simulink model "Bioloid_DFK_MDL_SV"  (R2013a)
settings: Solver=ode45  StartTime=0.0  StopTime=20  FixedStep=0.001  RelTol=1e-12
undefined symbols (not defined in the file or in its folder): Bioloid_DFK_SV, Bioloid_Ja_SV, Bioloid_Jg_SV, Bioloid_Signals2VRML, Error_Poses, ToSimulink_Bioloid_FK_ST
libraries: simulink x24, vrlib x1
settings Model: Creator=Jose Angel Rangel  LastModifiedBy=Angel

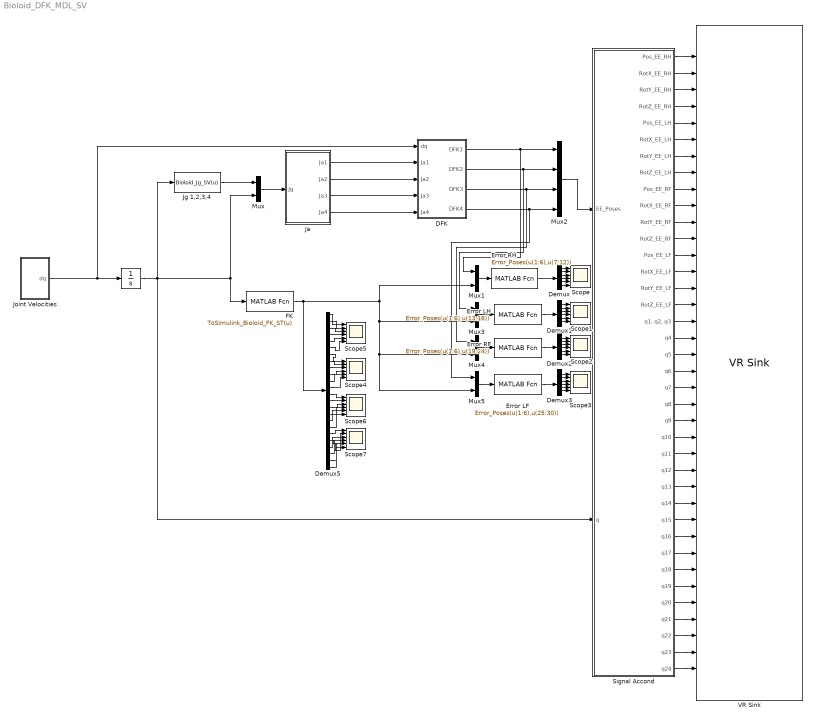
== system Bioloid_DFK_MDL_SV ==
  " " : Integrator
  DFK : Subsystem
  Demux{,1..3} (4 alike) : Demux  Outputs=6
  Demux5 : Demux  Outputs=24
  Error LF : MATLABFcn  MATLABFcn=Error_Poses(u(1:6),u(25:30))  OutputDimensions=6
  Error LH : MATLABFcn  MATLABFcn=Error_Poses(u(1:6),u(13:18))  OutputDimensions=6
  Error RF : MATLABFcn  MATLABFcn=Error_Poses(u(1:6),u(19:24))  OutputDimensions=6
  Error RH : MATLABFcn  MATLABFcn=Error_Poses(u(1:6),u(7:12))  OutputDimensions=6
  FK : MATLABFcn  MATLABFcn=ToSimulink_Bioloid_FK_ST(u)  OutputDimensions=24
  "Ja " : Subsystem
  Jg 1,2,3,4 : MATLABFcn  MATLABFcn=Bioloid_Jg_SV(u)  OutputDimensions=600
  Joint Velocities : Subsystem
  Mux{,1,3..5} (5 alike) : Mux  Inputs=2
  Mux2 : Mux
  Scope{,1..7} (8 alike) : Scope  NumInputPorts=6
      Scope settings: YMin=7e-10~1.03398e-25~0~-1~-1~-7e-06  YMax=1.7e-09~2.75e-09~6e-17~1~1~-1e-06
      Scope1 settings: TimeRange=10  YMin=-2.5e-05~-5e-06~-2e-05~-1~-0.007~-7  YMax=5e-06~3.5e-05~2.5e-06~7~0.001~1
      Scope2 settings: YMin=-7e-05~-0.000175~-2e-05~-5~-0.075~-3.5  YMax=1e-05~2.5e-05~6e-05~40~0.1~0.5  SaveName=ScopeData2
      Scope3 settings: YMin=-7e-05~-0.000175~-2e-05~-5~-0.075~-3.5  YMax=1e-05~2.5e-05~6e-05~40~0.1~0.5  SaveName=ScopeData3
      Scope4 settings: YMin=-2e-05~-9e-05~4e-05~0~-0.015~-7  YMax=7.5e-06~-2e-05~0.00011~7~-0.005~0  SaveName=ScopeData4
      Scope5 settings: YMin=4.6~4.6~4.9~-1.7~-0.015~-7  YMax=5.6~5.4~5.8~-0.7~-0.005~0  SaveName=ScopeData5
      Scope6 settings: YMin=-2e-05~-9e-05~4e-05~0~-0.015~-7  YMax=7.5e-06~-2e-05~0.00011~7~-0.005~0  SaveName=ScopeData6
      Scope7 settings: YMin=-2e-05~-9e-05~4e-05~0~-0.015~-7  YMax=7.5e-06~-2e-05~0.00011~7~-0.005~0  SaveName=ScopeData7
  Signal Accond : Subsystem
  VR Sink : vrlib/VR Sink  InstantiateOnLoad=on  SampleTime=0.1  ViewEnable=on  RemoteChange=off  RemoteView=off  FieldsWritten=EE_RH_Traslation.translation.3.1.1.double#EE_RH_RotX.rotation.4.1.1.double#EE_RH_RotY.rotation.4.1.1.double#EE_RH_RotZ.rotation.4.1.1.double#EE_LH_Traslation.translation.3.1.1.double#EE_LH_RotX.rotation.4.1.1.double#EE_LH_RotY.rotation.4.1.1.double#EE_LH_RotZ.rotation.4.1.1.double#EE_RF_Traslation.translation.3.1.1.double#EE_RF_RotX.rotation.4.1.1.double#EE_RF_RotY.rotation.4.1.1.double#EE_RF_RotZ.rotation.4.1.1.double#EE_LF_Traslation.translation.3.1.1.double#EE_LF_RotX.rotation.4.1.1.double#EE_LF_RotY.rotation.4.1.1.double#EE_LF_RotZ.rotation.4.1.1.double#TrunkTraslation.translation.3.1.1.double#TrunkRotX.rotation.4.1.1.double#TrunkRotY.rotation.4.1.1.double#TrunkRotZ.rotation.4.1.1.double#Right_Arm.rotation.4.1.1.double#Right_Humeros1.rotation.4.1.1.double#Right_Hand1.rotation.4.1.1.double#Left_Arm.rotation.4.1.1.double#Left_Humeros1.rotation.4.1.1.double#Left_Hand1.rotation.4.1.1.double#Right_Groin.rotation.4.1.1.double#Right_Hip1.rotation.4.1.1.double#Right_Femur1.rotation.4.1.1.double#Right_Tibia1.rotation.4.1.1.double#Right_Ankle1.rotation.4.1.1.double#Right_Foot1.rotation.4.1.1.double#Left_Groin.rotation.4.1.1.double#Left_Hip1.rotation.4.1.1.double#Left_Femur1.rotation.4.1.1.double#Left_Tibia1.rotation.4.1.1.double#Left_Ankle1.rotation.4.1.1.double#Left_Foot1.rotation.4.1.1.double  WorldFileName=Bioloid (Fisico White_Background).WRL  AutoView=off  VideoDimensions=[]  AllowVariableSize=off
  wires:
  Jg 1,2,3,4/1 -> Mux/1
  "Ja "/1(Ja1) -> DFK/2(Ja1)
  "Ja "/2(Ja2) -> DFK/3(Ja2)
  "Ja "/3(Ja3) -> DFK/4(Ja3)
  "Ja "/4(Ja4) -> DFK/5(Ja4)
  Joint Velocities/1(dq) -> DFK/1(dq), " "/1
  " "/1 -> Signal Accond/2(q), Mux/2, FK/1, Jg 1,2,3,4/1
  DFK/1(DFK1) -> Mux1/1, Mux2/1
  DFK/2(DFK2) -> Mux3/1, Mux2/2
  DFK/3(DFK3) -> Mux4/1, Mux2/3
  DFK/4(DFK4) -> Mux5/1, Mux2/4
  Demux/6 -> Scope/6
  Demux/3 -> Scope/3
  Demux/4 -> Scope/4
  Demux/5 -> Scope/5
  Demux/2 -> Scope/2
  Demux/1 -> Scope/1
  Demux1/6 -> Scope1/6
  Demux1/3 -> Scope1/3
  Demux1/4 -> Scope1/4
  Demux1/5 -> Scope1/5
  Demux1/2 -> Scope1/2
  Demux1/1 -> Scope1/1
  Demux2/6 -> Scope2/6
  Demux2/3 -> Scope2/3
  Demux2/4 -> Scope2/4
  Demux2/5 -> Scope2/5
  Demux2/2 -> Scope2/2
  Demux2/1 -> Scope2/1
  Demux3/6 -> Scope3/6
  Demux3/3 -> Scope3/3
  Demux3/4 -> Scope3/4
  Demux3/5 -> Scope3/5
  Demux3/2 -> Scope3/2
  Demux3/1 -> Scope3/1
  Mux1/1 -> Error RH/1
  Mux3/1 -> Error LH/1
  Mux4/1 -> Error RF/1
  Mux5/1 -> Error LF/1
  Error RH/1 -> Demux/1
  Mux/1 -> "Ja "/1(Jg)
  Error LH/1 -> Demux1/1
  Error RF/1 -> Demux2/1
  Error LF/1 -> Demux3/1
  Signal Accond/1(Pos_EE_RH) -> VR Sink/1
  Signal Accond/2(RotX_EE_RH) -> VR Sink/2
  Signal Accond/3(RotY_EE_RH) -> VR Sink/3
  Signal Accond/4(RotZ_EE_RH) -> VR Sink/4
  Signal Accond/5(Pos_EE_LH) -> VR Sink/5
  Signal Accond/30(q16) -> VR Sink/30
  Signal Accond/16(RotZ_EE_LF) -> VR Sink/16
  Signal Accond/36(q22) -> VR Sink/36
  Signal Accond/24(q10) -> VR Sink/24
  Signal Accond/22(q8) -> VR Sink/22
  Signal Accond/31(q17) -> VR Sink/31
  Signal Accond/20(q6) -> VR Sink/20
  Signal Accond/32(q18) -> VR Sink/32
  Signal Accond/21(q7) -> VR Sink/21
  Signal Accond/6(RotX_EE_LH) -> VR Sink/6
  Signal Accond/7(RotY_EE_LH) -> VR Sink/7
  Signal Accond/18(q4) -> VR Sink/18
  Signal Accond/25(q11) -> VR Sink/25
  Signal Accond/26(q12) -> VR Sink/26
  Signal Accond/15(RotY_EE_LF) -> VR Sink/15
  Signal Accond/38(q24) -> VR Sink/38
  Signal Accond/17("q1, q2, q3") -> VR Sink/17
  Signal Accond/29(q15) -> VR Sink/29
  Signal Accond/9(Pos_EE_RF) -> VR Sink/9
  Signal Accond/27(q13) -> VR Sink/27
  Signal Accond/10(RotX_EE_RF) -> VR Sink/10
  Signal Accond/12(RotZ_EE_RF) -> VR Sink/12
  Signal Accond/8(RotZ_EE_LH) -> VR Sink/8
  Signal Accond/19("q5 ") -> VR Sink/19
  Signal Accond/13(Pos_EE_LF) -> VR Sink/13
  Signal Accond/33(q19) -> VR Sink/33
  Signal Accond/35(q21) -> VR Sink/35
  Signal Accond/11(RotY_EE_RF) -> VR Sink/11
  Signal Accond/34(q20) -> VR Sink/34
  Signal Accond/14(RotX_EE_LF) -> VR Sink/14
  Signal Accond/23(q9) -> VR Sink/23
  Signal Accond/28(q14) -> VR Sink/28
  Signal Accond/37(q23) -> VR Sink/37
  Mux2/1 -> Signal Accond/1(EE_Poses)
  FK/1 -> Demux5/1, Mux3/2, Mux5/2, Mux4/2, Mux1/2
  Demux5/1 -> Scope5/1
  Demux5/2 -> Scope5/2
  Demux5/3 -> Scope5/3
  Demux5/4 -> Scope5/4
  Demux5/5 -> Scope5/5
  Demux5/6 -> Scope5/6
  Demux5/7 -> Scope4/1
  Demux5/8 -> Scope4/2
  Demux5/9 -> Scope4/3
  Demux5/10 -> Scope4/4
  Demux5/11 -> Scope4/5
  Demux5/12 -> Scope4/6
  Demux5/13 -> Scope6/1
  Demux5/14 -> Scope6/2
  Demux5/15 -> Scope6/3
  Demux5/16 -> Scope6/4
  Demux5/17 -> Scope6/5
  Demux5/18 -> Scope6/6
  Demux5/19 -> Scope7/1
  Demux5/20 -> Scope7/2
  Demux5/21 -> Scope7/3
  Demux5/22 -> Scope7/4
  Demux5/23 -> Scope7/5
  Demux5/24 -> Scope7/6

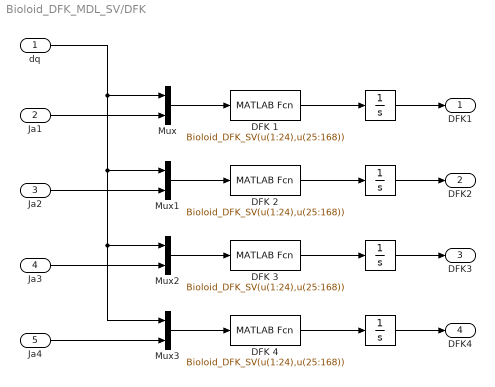
== system Bioloid_DFK_MDL_SV/DFK ==
  dq : Inport
  Ja1 : Inport  Port=2
  Ja2 : Inport  Port=3
  Ja3 : Inport  Port=4
  Ja4 : Inport  Port=5
  "  " : Integrator  InitialCondition=[0;-0.2250;-0.0145;0;0;0]
  "    " : Integrator  InitialCondition=[0;0.225;-0.0145;0;0;0]
  "     " : Integrator  InitialCondition=[0;-0.0385;-0.30250;0;0;0]
  "      " : Integrator  InitialCondition=[0;0.0385;-0.3025;0;0;0]
  DFK {1..4} (4 alike) : MATLABFcn  MATLABFcn=Bioloid_DFK_SV(u(1:24),u(25:168))  OutputDimensions=6
  Mux{,1..3} (4 alike) : Mux  Inputs=2
  DFK1 : Outport
  DFK2 : Outport  Port=2
  DFK3 : Outport  Port=3
  DFK4 : Outport  Port=4
  wires:
  DFK 1/1 -> "  "/1
  DFK 2/1 -> "    "/1
  DFK 3/1 -> "     "/1
  DFK 4/1 -> "      "/1
  dq/1 -> Mux3/1, Mux2/1, Mux1/1, Mux/1
  Mux/1 -> DFK 1/1
  Mux1/1 -> DFK 2/1
  Mux2/1 -> DFK 3/1
  Mux3/1 -> DFK 4/1
  Ja1/1 -> Mux/2
  Ja2/1 -> Mux1/2
  Ja3/1 -> Mux2/2
  Ja4/1 -> Mux3/2
  "  "/1 -> DFK1/1
  "    "/1 -> DFK2/1
  "     "/1 -> DFK3/1
  "      "/1 -> DFK4/1

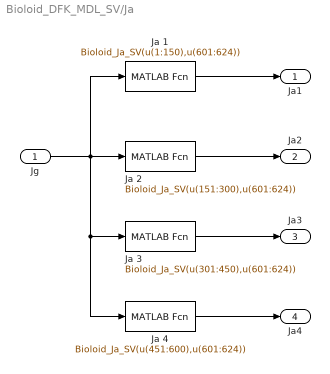
== system Bioloid_DFK_MDL_SV/Ja  ==
  Jg : Inport
  Ja 1 : MATLABFcn  MATLABFcn=Bioloid_Ja_SV(u(1:150),u(601:624))  OutputDimensions=144
  Ja 2 : MATLABFcn  MATLABFcn=Bioloid_Ja_SV(u(151:300),u(601:624))  OutputDimensions=144
  Ja 3 : MATLABFcn  MATLABFcn=Bioloid_Ja_SV(u(301:450),u(601:624))  OutputDimensions=144
  Ja 4 : MATLABFcn  MATLABFcn=Bioloid_Ja_SV(u(451:600),u(601:624))  OutputDimensions=144
  Ja1 : Outport
  Ja2 : Outport  Port=2
  Ja3 : Outport  Port=3
  Ja4 : Outport  Port=4
  wires:
  Jg/1 -> Ja 1/1, Ja 2/1, Ja 3/1, Ja 4/1
  Ja 4/1 -> Ja4/1
  Ja 1/1 -> Ja1/1
  Ja 3/1 -> Ja3/1
  Ja 2/1 -> Ja2/1

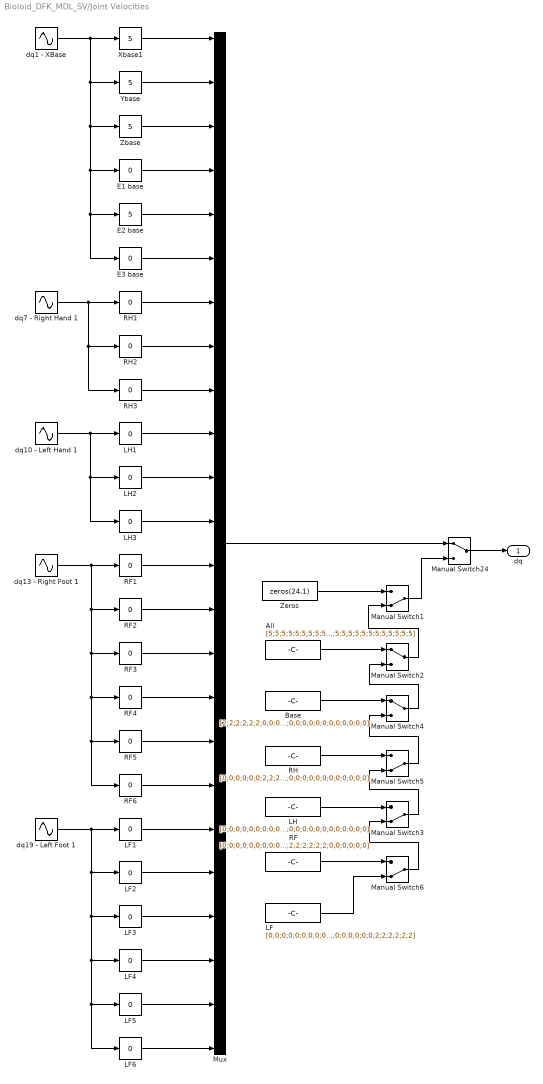
== system Bioloid_DFK_MDL_SV/Joint Velocities ==
  All : Constant  Value=[5;5;5;5;5;5;5;5;5;5;5;5;5;5;5;5;5;5;5;5;5;5;5;5]
  Base : Constant  Value=[2;2;2;2;2;2;0;0;0;0;0;0;0;0;0;0;0;0;0;0;0;0;0;0]
  E1 base : simulink/Math Operations/Slider Gain  low=-5  gain=0  high=5
  E2 base : simulink/Math Operations/Slider Gain  low=-5  gain=5  high=5
  E3 base : simulink/Math Operations/Slider Gain  low=-5  gain=0  high=5
  LF : Constant  Value=[0;0;0;0;0;0;0;0;0;0;0;0;0;0;0;0;0;0;2;2;2;2;2;2]
  LF{1..6} (6 alike) : simulink/Math Operations/Slider Gain  low=0  gain=0  high=5
  LH : Constant  Value=[0;0;0;0;0;0;0;0;0;2;2;2;0;0;0;0;0;0;0;0;0;0;0;0]
  LH1 : simulink/Math Operations/Slider Gain  low=0  gain=0  high=5
  LH2 : simulink/Math Operations/Slider Gain  low=0  gain=0  high=5
  LH3 : simulink/Math Operations/Slider Gain  low=0  gain=0  high=5
  Manual Switch{1,3,5..6} (4 alike) : ManualSwitch  CurrentSetting=0
  Manual Switch2 : ManualSwitch
  Manual Switch24 : ManualSwitch
  Manual Switch4 : ManualSwitch
  Mux : Mux  Inputs=24
  RF : Constant  Value=[0;0;0;0;0;0;0;0;0;0;0;0;2;2;2;2;2;2;0;0;0;0;0;0]
  RF{1..6} (6 alike) : simulink/Math Operations/Slider Gain  low=0  gain=0  high=5
  RH : Constant  Value=[0;0;0;0;0;0;2;2;2;0;0;0;0;0;0;0;0;0;0;0;0;0;0;0]
  RH1 : simulink/Math Operations/Slider Gain  low=0  gain=0  high=5
  RH2 : simulink/Math Operations/Slider Gain  low=0  gain=0  high=5
  RH3 : simulink/Math Operations/Slider Gain  low=0  gain=0  high=5
  Xbase1 : simulink/Math Operations/Slider Gain  low=-5  gain=5  high=5
  Ybase : simulink/Math Operations/Slider Gain  low=-5  gain=5  high=5
  Zbase : simulink/Math Operations/Slider Gain  low=-5  gain=5  high=5
  Zeros : Constant  Value=zeros(24,1)
  dq1 - XBase : Sin  SampleTime=0
  dq10 - Left Hand 1 : Sin  SampleTime=0
  dq13 - Right Foot 1 : Sin  SampleTime=0
  dq19 - Left Foot 1 : Sin  SampleTime=0
  dq7 - Right Hand 1 : Sin  SampleTime=0
  dq : Outport
  wires:
  Mux/1 -> Manual Switch24/1
  Manual Switch24/1 -> dq/1
  dq19 - Left Foot 1/1 -> LF3/1, LF6/1, LF5/1, LF4/1, LF2/1, LF1/1
  dq13 - Right Foot 1/1 -> RF2/1, RF3/1, RF4/1, RF5/1, RF6/1, RF1/1
  dq7 - Right Hand 1/1 -> RH3/1, RH2/1, RH1/1
  E1 base/1 -> Mux/4
  E2 base/1 -> Mux/5
  E3 base/1 -> Mux/6
  Zbase/1 -> Mux/3
  RH1/1 -> Mux/7
  RH2/1 -> Mux/8
  RH3/1 -> Mux/9
  LH1/1 -> Mux/10
  LH2/1 -> Mux/11
  LH3/1 -> Mux/12
  RF4/1 -> Mux/16
  RF5/1 -> Mux/17
  RF6/1 -> Mux/18
  RF1/1 -> Mux/13
  RF2/1 -> Mux/14
  RF3/1 -> Mux/15
  LF1/1 -> Mux/19
  LF2/1 -> Mux/20
  LF3/1 -> Mux/21
  LF4/1 -> Mux/22
  LF5/1 -> Mux/23
  LF6/1 -> Mux/24
  dq1 - XBase/1 -> Ybase/1, Zbase/1, E1 base/1, E2 base/1, E3 base/1, Xbase1/1
  Ybase/1 -> Mux/2
  Xbase1/1 -> Mux/1
  dq10 - Left Hand 1/1 -> LH3/1, LH2/1, LH1/1
  Manual Switch1/1 -> Manual Switch24/2
  Zeros/1 -> Manual Switch1/1
  Manual Switch2/1 -> Manual Switch1/2
  All/1 -> Manual Switch2/1
  Manual Switch4/1 -> Manual Switch2/2
  Base/1 -> Manual Switch4/1
  Manual Switch5/1 -> Manual Switch4/2
  RH/1 -> Manual Switch5/1
  Manual Switch3/1 -> Manual Switch5/2
  LH/1 -> Manual Switch3/1
  Manual Switch6/1 -> Manual Switch3/2
  RF/1 -> Manual Switch6/1
  LF/1 -> Manual Switch6/2

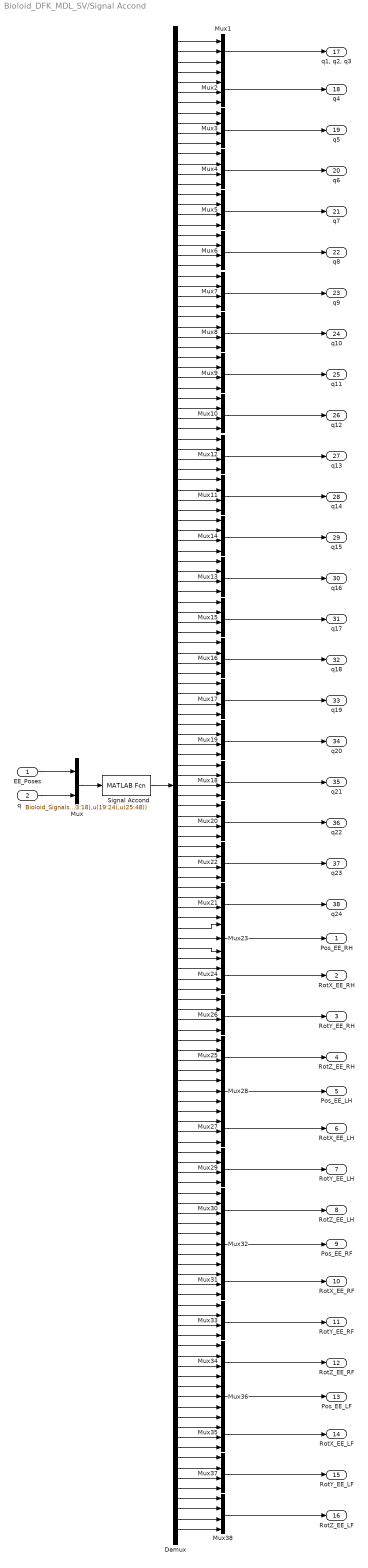
== system Bioloid_DFK_MDL_SV/Signal Accond ==
  EE_Poses : Inport
  q : Inport  Port=2
  Demux : Demux  Outputs=147
  Mux : Mux  Inputs=2
  Mux{1,23,28,32,36} (5 alike) : Mux  Inputs=3
  Mux{2..22,24..27,29..31,33..35,37..38} (33 alike) : Mux
  Signal Accond : MATLABFcn  MATLABFcn=Bioloid_Signals2VRML(u(1:6),u(7:12),u(13:18),u(19:24),u(25:48))
  Pos_EE_RH : Outport
  RotX_EE_RH : Outport  Port=2
  RotY_EE_RH : Outport  Port=3
  RotZ_EE_RH : Outport  Port=4
  Pos_EE_LH : Outport  Port=5
  RotX_EE_LH : Outport  Port=6
  RotY_EE_LH : Outport  Port=7
  RotZ_EE_LH : Outport  Port=8
  Pos_EE_RF : Outport  Port=9
  RotX_EE_RF : Outport  Port=10
  RotY_EE_RF : Outport  Port=11
  RotZ_EE_RF : Outport  Port=12
  Pos_EE_LF : Outport  Port=13
  RotX_EE_LF : Outport  Port=14
  RotY_EE_LF : Outport  Port=15
  RotZ_EE_LF : Outport  Port=16
  "q1, q2, q3" : Outport  Port=17
  q4 : Outport  Port=18
  "q5 " : Outport  Port=19
  q6 : Outport  Port=20
  q7 : Outport  Port=21
  q8 : Outport  Port=22
  q9 : Outport  Port=23
  q10 : Outport  Port=24
  q11 : Outport  Port=25
  q12 : Outport  Port=26
  q13 : Outport  Port=27
  q14 : Outport  Port=28
  q15 : Outport  Port=29
  q16 : Outport  Port=30
  q17 : Outport  Port=31
  q18 : Outport  Port=32
  q19 : Outport  Port=33
  q20 : Outport  Port=34
  q21 : Outport  Port=35
  q22 : Outport  Port=36
  q23 : Outport  Port=37
  q24 : Outport  Port=38
  wires:
  q/1 -> Mux/2
  EE_Poses/1 -> Mux/1
  Mux/1 -> Signal Accond/1
  Demux/7 -> Mux2/4
  Mux11/1 -> q14/1
  Demux/4 -> Mux2/1
  Mux38/1 -> RotZ_EE_LF/1
  Mux10/1 -> q12/1
  Demux/1 -> Mux1/1
  Demux/3 -> Mux1/3
  Mux18/1 -> q21/1
  Demux/6 -> Mux2/3
  Mux1/1 -> "q1, q2, q3"/1
  Mux15/1 -> q17/1
  Mux8/1 -> q10/1
  Demux/5 -> Mux2/2
  Demux/2 -> Mux1/2
  Demux/8 -> Mux3/1
  Mux28/1 -> Pos_EE_LH/1
  Mux16/1 -> q18/1
  Mux3/1 -> "q5 "/1
  Mux7/1 -> q9/1
  Mux14/1 -> q15/1
  Mux9/1 -> q11/1
  Mux22/1 -> q23/1
  Mux2/1 -> q4/1
  Mux4/1 -> q6/1
  Mux5/1 -> q7/1
  Mux30/1 -> RotZ_EE_LH/1
  Mux13/1 -> q16/1
  Mux12/1 -> q13/1
  Mux24/1 -> RotX_EE_RH/1
  Mux20/1 -> q22/1
  Mux19/1 -> q20/1
  Mux6/1 -> q8/1
  Mux25/1 -> RotZ_EE_RH/1
  Mux17/1 -> q19/1
  Mux26/1 -> RotY_EE_RH/1
  Mux21/1 -> q24/1
  Mux23/1 -> Pos_EE_RH/1
  Mux36/1 -> Pos_EE_LF/1
  Mux32/1 -> Pos_EE_RF/1
  Mux31/1 -> RotX_EE_RF/1
  Mux33/1 -> RotY_EE_RF/1
  Mux35/1 -> RotX_EE_LF/1
  Mux34/1 -> RotZ_EE_RF/1
  Mux37/1 -> RotY_EE_LF/1
  Mux27/1 -> RotX_EE_LH/1
  Mux29/1 -> RotY_EE_LH/1
  Demux/10 -> Mux3/3
  Demux/9 -> Mux3/2
  Demux/11 -> Mux3/4
  Demux/12 -> Mux4/1
  Demux/15 -> Mux4/4
  Demux/13 -> Mux4/2
  Demux/14 -> Mux4/3
  Signal Accond/1 -> Demux/1
  Demux/55 -> Mux13/4
  Demux/50 -> Mux14/3
  Demux/70 -> Mux19/3
  Demux/45 -> Mux11/2
  Demux/37 -> Mux10/2
  Demux/28 -> Mux8/1
  Demux/35 -> Mux9/4
  Demux/40 -> Mux12/1
  Demux/27 -> Mux7/4
  Demux/41 -> Mux12/2
  Demux/46 -> Mux11/3
  Demux/69 -> Mux19/2
  Demux/58 -> Mux15/3
  Demux/33 -> Mux9/2
  Demux/20 -> Mux6/1
  Demux/66 -> Mux17/3
  Demux/36 -> Mux10/1
  Demux/26 -> Mux7/3
  Demux/59 -> Mux15/4
  Demux/49 -> Mux14/2
  Demux/47 -> Mux11/4
  Demux/60 -> Mux16/1
  Demux/38 -> Mux10/3
  Demux/63 -> Mux16/4
  Demux/54 -> Mux13/3
  Demux/18 -> Mux5/3
  Demux/34 -> Mux9/3
  Demux/44 -> Mux11/1
  Demux/29 -> Mux8/2
  Demux/51 -> Mux14/4
  Demux/31 -> Mux8/4
  Demux/30 -> Mux8/3
  Demux/64 -> Mux17/1
  Demux/16 -> Mux5/1
  Demux/53 -> Mux13/2
  Demux/52 -> Mux13/1
  Demux/17 -> Mux5/2
  Demux/22 -> Mux6/3
  Demux/48 -> Mux14/1
  Demux/43 -> Mux12/4
  Demux/25 -> Mux7/2
  Demux/24 -> Mux7/1
  Demux/32 -> Mux9/1
  Demux/56 -> Mux15/1
  Demux/39 -> Mux10/4
  Demux/23 -> Mux6/4
  Demux/21 -> Mux6/2
  Demux/61 -> Mux16/2
  Demux/19 -> Mux5/4
  Demux/42 -> Mux12/3
  Demux/67 -> Mux17/4
  Demux/65 -> Mux17/2
  Demux/57 -> Mux15/2
  Demux/62 -> Mux16/3
  Demux/68 -> Mux19/1
  Demux/113 -> Mux29/4
  Demux/86 -> Mux21/3
  Demux/143 -> Mux37/4
  Demux/107 -> Mux27/2
  Demux/112 -> Mux29/3
  Demux/131 -> Mux34/3
  Demux/133 -> Mux36/1
  Demux/126 -> Mux33/2
  Demux/139 -> Mux35/4
  Demux/83 -> Mux22/4
  Demux/72 -> Mux18/1
  Demux/134 -> Mux36/2
  Demux/137 -> Mux35/2
  Demux/115 -> Mux30/2
  Demux/132 -> Mux34/4
  Demux/125 -> Mux33/1
  Demux/71 -> Mux19/4
  Demux/89 -> Mux23/2
  Demux/128 -> Mux33/4
  Demux/144 -> Mux38/1
  Demux/77 -> Mux20/2
  Demux/118 -> Mux32/1
  Demux/103 -> Mux28/1
  Demux/101 -> Mux25/3
  Demux/100 -> Mux25/2
  Demux/78 -> Mux20/3
  Demux/98 -> Mux26/4
  Demux/142 -> Mux37/3
  Demux/102 -> Mux25/4
  Demux/138 -> Mux35/3
  Demux/123 -> Mux31/3
  Demux/96 -> Mux26/2
  Demux/145 -> Mux38/2
  Demux/99 -> Mux25/1
  Demux/122 -> Mux31/2
  Demux/84 -> Mux21/1
  Demux/116 -> Mux30/3
  Demux/114 -> Mux30/1
  Demux/88 -> Mux23/1
  Demux/108 -> Mux27/3
  Demux/121 -> Mux31/1
  Demux/120 -> Mux32/3
  Demux/76 -> Mux20/1
  Demux/90 -> Mux23/3
  Demux/147 -> Mux38/4
  Demux/111 -> Mux29/2
  Demux/85 -> Mux21/2
  Demux/79 -> Mux20/4
  Demux/93 -> Mux24/3
  Demux/74 -> Mux18/3
  Demux/109 -> Mux27/4
  Demux/136 -> Mux35/1
  Demux/87 -> Mux21/4
  Demux/127 -> Mux33/3
  Demux/82 -> Mux22/3
  Demux/146 -> Mux38/3
  Demux/80 -> Mux22/1
  Demux/81 -> Mux22/2
  Demux/75 -> Mux18/4
  Demux/97 -> Mux26/3
  Demux/91 -> Mux24/1
  Demux/95 -> Mux26/1
  Demux/124 -> Mux31/4
  Demux/105 -> Mux28/3
  Demux/73 -> Mux18/2
  Demux/104 -> Mux28/2
  Demux/94 -> Mux24/4
  Demux/92 -> Mux24/2
  Demux/135 -> Mux36/3
  Demux/110 -> Mux29/1
  Demux/130 -> Mux34/2
  Demux/140 -> Mux37/1
  Demux/141 -> Mux37/2
  Demux/117 -> Mux30/4
  Demux/129 -> Mux34/1
  Demux/119 -> Mux32/2
  Demux/106 -> Mux27/1
